simulink model "TesteMobotic_Initialization"  (R2024a)
settings: Solver=FixedStepDiscrete  StartTime=0.0  StopTime=inf  FixedStep=1e-3  RelTol=1e-3
model workspace (MAT data in the model file):
  RTK_health_condition = 30
  mdlWSDbList = ["tramontina_database_curtis.dbc" "tramontina_database_curtis_mesa.dbc" "tramontina_database_mobotic.dbc" "tramontina_database_nvidia.dbc" "tramontina_database_sick_modbus.dbc" "tramontina_database_xsens.dbc"]
undefined symbols (not defined in the file): Down, Pull
libraries: speedgoatlib_IO60X_IO69X x6, tramontina_database_curtislib x5, tramontina_database_curtis_mesalib x2, tramontina_database_moboticlib x2, speedgoatlib_IO691 x2, tramontina_database_nvidialib x1, canmsglib x1
settings Model: DataDictionary=configuration_dictionary.sldd  SimulationMode=external  ExtModeEnableFloating=off  Creator=matlab.cut  LastModifiedBy=matlab.cut
settings SolverCC: ConcurrentTasks=on  PositivePriorityOrder=on
settings OptimizationCC: BlockReduction=off  DefaultParameterBehavior=Inlined  OptimizeBlockIOStorage=off  EnhancedBackFolding=on  PassReuseOutputArgsThreshold=0  OptimizeBlockOrder=speed  DifferentSizesBufferReuse=on
settings DebuggingCC: UnderspecifiedInitializationDetection=Classic  MergeDetectMultiDrivingBlocksExec=none  TasksWithSamePriorityMsg=none  ParameterTunabilityLossMsg=error
settings HardwareCC: ProdBitPerLong=64  ProdLongLongMode=on  ProdHWDeviceType=Intel->x86-64 (Linux 64)
settings ModelReferenceCC: PropagateSignalLabelsOutOfModel=off
settings SFSimCC: MATLABDynamicMemAlloc=off
settings RTWCC: Description=Speedgoat Real-Time Target Machine  SystemTargetFile=speedgoat.tlc  TemplateMakefile=slrealtime_default_tmf  Toolchain=Simulink Real-Time Toolchain  BuildConfiguration=Faster Runs  CodeExecutionProfiling=on  TargetLang=C++  GPUComputeCapability=3.5
settings CodeAppCC: ForceParamTrailComments=on  MaxIdLength=127  OperatorAnnotations=on
settings SimulinkRealTimeTargetCC: InstructionSetFMA=off  LogToMDFFile=off

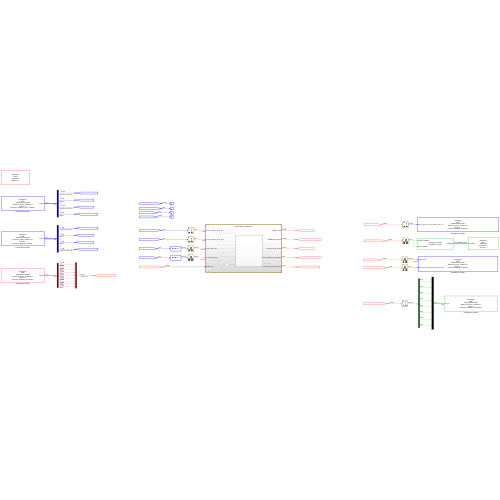
[thumbnail: Simulink's stored preview of the top-level diagram]
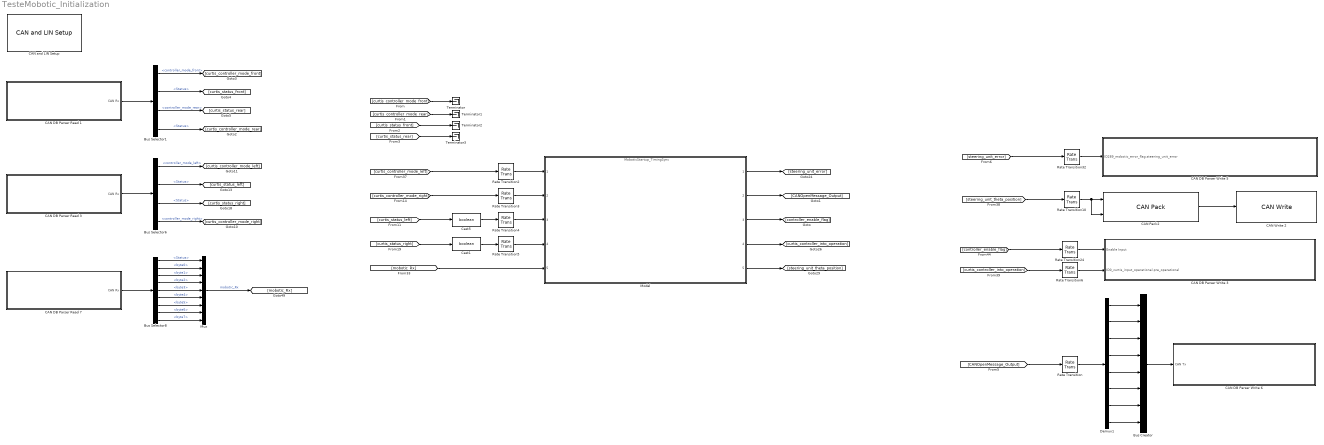
== system TesteMobotic_Initialization ==
  Bus Creator : BusCreator  Inputs=8
  Bus Selector1 : BusSelector  OutputSignals=ID1832_controller_status_RCUfront.controller_mode_front,ID1832_controller_status_RCUfront.MessageStatus.Status,ID1833_controller_status_RCUrear.controller_mode_rear,ID1833_controller_status_RCUrear.MessageStatus.Status
  Bus Selector6 : BusSelector  OutputSignals=ID1830_controller_status_left.controller_mode_left,ID1830_controller_status_left.MessageStatus.Status,ID1831_controller_status_right.MessageStatus.Status,ID1831_controller_status_right.controller_mode_right
  Bus Selector8 : BusSelector  OutputSignals=ID1459_feedback_word.MessageStatus.Status,ID1459_feedback_word.byte0,ID1459_feedback_word.byte1,ID1459_feedback_word.byte2,ID1459_feedback_word.byte3,ID1459_feedback_word.byte4,ID1459_feedback_word.byte5,ID1459_feedback_word.byte6,ID1459_feedback_word.byte7
  CAN DB Parser Read 1 : Subsystem
      settings: OpenFcn=sg_can.OpenFcnRead;
      mask Help: eval('sg.utils.help.show(''io_main/refentry_ref_can_ofa_parsing_read'');')
      mask Display: disp('Speedgoat\nIO691\nCAN DB Parser Read\nModule ID: IO691 - Module ID 1\nChannel:  1\ntramontina_database_curtis_mesa.dbc ');
  CAN DB Parser Read 3 : Subsystem
      settings: OpenFcn=sg_can.OpenFcnRead;
      mask Help: eval('sg.utils.help.show(''io_main/refentry_ref_can_ofa_parsing_read'');')
      mask Display: disp('Speedgoat\nIO691\nCAN DB Parser Read\nModule ID: IO691 - Module ID 1\nChannel:  1\ntramontina_database_curtis.dbc ');
  CAN DB Parser Read 7 : Subsystem
      settings: OpenFcn=sg_can.OpenFcnRead;
      mask Help: eval('sg.utils.help.show(''io_main/refentry_ref_can_ofa_parsing_read'');')
      mask Display: disp('Speedgoat\nIO691\nCAN DB Parser Read\nModule ID: IO691 - Module ID 1\nChannel:  1\ntramontina_database_mobotic.dbc ');
  CAN DB Parser Write 3 : Subsystem
      settings: OpenFcn=sg_can.OpenFcnWrite;
      mask Help: eval('sg.utils.help.show(''io_main/refentry_ref_can_ofa_parsing_write'');')
      mask Display: disp('Speedgoat\nIO691\nCAN DB Parser Write\nModule ID: IO691 - Module ID 1\nChannel:  1\ntramontina_database_curtis.dbc ');
  CAN DB Parser Write 5 : Subsystem
      settings: OpenFcn=sg_can.OpenFcnWrite;
      mask Help: eval('sg.utils.help.show(''io_main/refentry_ref_can_ofa_parsing_write'');')
      mask Display: disp('Speedgoat\nIO691\nCAN DB Parser Write\nModule ID: IO691 - Module ID 1\nChannel:  1\ntramontina_database_nvidia.dbc ');
  CAN DB Parser Write 6 : Subsystem
      settings: OpenFcn=sg_can.OpenFcnWrite;
      mask Help: eval('sg.utils.help.show(''io_main/refentry_ref_can_ofa_parsing_write'');')
      mask Display: disp('Speedgoat\nIO691\nCAN DB Parser Write\nModule ID: IO691 - Module ID 1\nChannel:  1\ntramontina_database_mobotic.dbc ');
  CAN Pack2 : canmsglib/CAN Pack  MsgList=(none)  MsgName=CAN Msg  MsgIDType=Standard (11-bit identifier)  MsgIdentifier=0x120  MsgLength=8  Remote=off  ApplyMinMax=off  BusOutput=on  SignalInfo={ 'position_feedback', '0', '32', 'LE', 'signed', 'Standard', '0', '1', '0', '-inf', 'inf'; 'pulse_feedback', '32', '32', 'LE', 'signed', 'Standard', '0', '1', '0', '-Inf', 'Inf' }
      settings: DataFormat=manually specified signals
  CAN Write 2 : speedgoatlib_IO691/CAN Write   moduleType=IO691  id=1  channel=1  canType=CAN (HS)  messageType=CAN (HS)  useBusIn=on  numOfMsg=1  enableInput=off  enableStatusPort=off  ts=10e-3  initValues=[691 1 0.01 0 1 1 0 1 0 1]
      settings: SourceProductName=IO691
  "CAN and LIN Setup " : speedgoatlib_IO691/CAN and LIN Setup   moduleInitValues="[691    1    1   -1   -1]"  id=1  moduleType=IO691  pciSlot=-1  canChn1=CAN (HS)  canChn2=Disabled  canChn3=Disabled  canChn4=Disabled  linChn1=Disabled  linChn2=Disabled  canInitStructArray=[]  canTermStructArray=[]  gpioChnx=Disabled  canChn1InitValues="[2   2   8   1  16   3  19   2   2   5   2   0]"  arbBdrChn1=500 kBaud  clockDividerChn1=Enable  arbManBdrChn1=[8,1,16,3]  fdBdrChn1=5.0 MBaud  fdManBdrChn1=[2,2,5,2]  termResistor1=off  canChn2InitValues="[1   0   2   8  31   8  19   2   2   5   2   0]"  arbBdrChn2=1.0 MBaud  clockDividerChn2=Enable  arbManBdrChn2=[2,8,31,8]  fdBdrChn2=5.0 MBaud  fdManBdrChn2=[2,2,5,2]  termResistor2=off  canChn3InitValues="[1   0   2   8  31   8  19   2   2   5   2   0]"  arbBdrChn3=1.0 MBaud  clockDividerChn3=Enable  arbManBdrChn3=[2,8,31,8]  fdBdrChn3=5.0 MBaud  fdManBdrChn3=[2,2,5,2]  termResistor3=off  canChn4InitValues="[1   0   2   8  31   8  19   2   2   5   2   0]"  arbBdrChn4=1.0 MBaud  clockDividerChn4=Enable  arbManBdrChn4=[2,8,31,8]  fdBdrChn4=5.0 MBaud  fdManBdrChn4=[2,2,5,2]  termResistor4=off  linChn1InitValues="[0  9600]"  linBtrChn1=9600  linChn2InitValues="[0  9600]"  linBtrChn2=9600  doInitTermStruct="[0  5  0  0  0]"  parDoChannels=[1 2]  parDoVoltage=5  parDoInitValues=0  parDoReset=1  parNumOfDoS=0  parDiChannels=[3 4]  parDiVoltage=5  parDiPull=Pull-Down
      settings: LibrarySourceBlock=speedgoatlib_IO602_IO691/CAN and LIN Setup
  Cast1 : DataTypeConversion  OutDataTypeStr=boolean  SaturateOnIntegerOverflow=off  RndMeth=Floor
  Cast5 : DataTypeConversion  OutDataTypeStr=boolean  SaturateOnIntegerOverflow=off  RndMeth=Floor
  Demux1 : Demux  Outputs=8
  Model : ModelReference  ModelNameDialog=MoboticStartup_TimingSync.slx  SimulationMode=Normal  ModelReferenceVersion=1.51
  Mux : Mux  Inputs=9
  Rate Transition{,2,6,10,24,32} (6 alike) : RateTransition
  Rate Transition3 : RateTransition  OutPortSampleTimeOpt=Inherit
  Rate Transition4 : RateTransition  OutPortSampleTimeOpt=Inherit
  Rate Transition5 : RateTransition  OutPortSampleTimeOpt=Inherit
  Terminator{,1..3} (4 alike) : Terminator
  wires:
  CAN Pack2/1 -> CAN Write 2/1
  Rate Transition6/1 -> CAN DB Parser Write 3/2(ID0_curtis_input_operational.pre_operational)
  [steering_unit_error] -> Rate Transition32/1
  Rate Transition10/1 -> CAN Pack2/2, CAN Pack2/1
  [curtis_controller_into_operation] -> Rate Transition6/1
  [steering_unit_theta_position] -> Rate Transition10/1
  [controller_enable_flag] -> Rate Transition24/1
  Rate Transition24/1 -> CAN DB Parser Write 3/1(Enable Input)
  Bus Selector6/2 -> [curtis_status_left]  "<Status>"
  Bus Selector8/7 -> Mux/7  "<byte5>"
  Bus Selector8/5 -> Mux/5  "<byte3>"
  Bus Selector8/1 -> Mux/1  "<Status>"
  Bus Selector8/2 -> Mux/2  "<byte0>"
  CAN DB Parser Read 3/1(CAN Rx) -> Bus Selector6/1
  CAN DB Parser Read 7/1(CAN Rx) -> Bus Selector8/1
  Bus Selector8/3 -> Mux/3  "<byte1>"
  Bus Selector8/6 -> Mux/6  "<byte4>"
  Mux/1 -> [mobotic_Rx]  "mobotic_Rx"
  Bus Selector8/8 -> Mux/8  "<byte6>"
  Bus Selector8/9 -> Mux/9  "<byte7>"
  Bus Selector6/4 -> [curtis_controller_mode_right]  "<controller_mode_right>"
  Bus Selector6/3 -> [curtis_status_right]  "<Status>"
  Bus Selector8/4 -> Mux/4  "<byte2>"
  Bus Selector6/1 -> [curtis_controller_mode_left]  "<controller_mode_left>"
  [curtis_controller_mode_left] -> Rate Transition2/1
  Cast5/1 -> Rate Transition4/1
  Cast1/1 -> Rate Transition5/1
  [curtis_controller_mode_right] -> Rate Transition3/1
  [curtis_status_left] -> Cast5/1
  [curtis_status_right] -> Cast1/1
  Rate Transition2/1 -> Model/1
  Rate Transition3/1 -> Model/2
  Rate Transition4/1 -> Model/3
  Rate Transition5/1 -> Model/4
  Rate Transition/1 -> Demux1/1
  Rate Transition32/1 -> CAN DB Parser Write 5/1(ID289_mobotic_error_flag.steering_unit_error)
  Model/2 -> [CANOpenMessage_Output]
  Model/1 -> [steering_unit_error]
  Model/5 -> [steering_unit_theta_position]
  Model/4 -> [curtis_controller_into_operation]
  Model/3 -> [controller_enable_flag]
  [CANOpenMessage_Output] -> Rate Transition/1
  Bus Selector1/1 -> [curtis_controller_mode_front]  "<controller_mode_front>"
  Bus Selector1/3 -> [curtis_status_rear]  "<controller_mode_rear>"
  Bus Selector1/4 -> [curtis_controller_mode_rear]  "<Status>"
  CAN DB Parser Read 1/1(CAN Rx) -> Bus Selector1/1
  Bus Selector1/2 -> [curtis_status_front]  "<Status>"
  [curtis_controller_mode_front] -> Terminator/1
  [curtis_status_front] -> Terminator2/1
  [curtis_controller_mode_rear] -> Terminator1/1
  [curtis_status_rear] -> Terminator3/1
  [mobotic_Rx] -> Model/5
  Demux1/1 -> Bus Creator/1
  Demux1/2 -> Bus Creator/2
  Demux1/3 -> Bus Creator/3
  Demux1/4 -> Bus Creator/4
  Demux1/5 -> Bus Creator/5
  Demux1/6 -> Bus Creator/6
  Demux1/7 -> Bus Creator/7
  Demux1/8 -> Bus Creator/8
  Bus Creator/1 -> CAN DB Parser Write 6/1(CAN Tx)

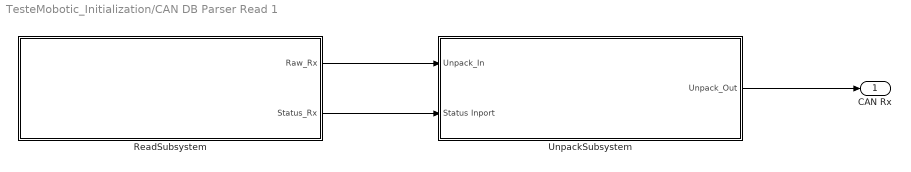
== system TesteMobotic_Initialization/CAN DB Parser Read 1 ==
  ReadSubsystem : Subsystem
  UnpackSubsystem : Subsystem
  CAN Rx : Outport
  wires:
  ReadSubsystem/1(Raw_Rx) -> UnpackSubsystem/1(Unpack_In)
  ReadSubsystem/2(Status_Rx) -> UnpackSubsystem/2(Status Inport)
  UnpackSubsystem/1(Unpack_Out) -> CAN Rx/1

== system TesteMobotic_Initialization/CAN DB Parser Read 3 ==
  ReadSubsystem : Subsystem
  UnpackSubsystem : Subsystem
  CAN Rx : Outport
  wires:
  ReadSubsystem/1(Raw_Rx) -> UnpackSubsystem/1(Unpack_In)
  ReadSubsystem/2(Status_Rx) -> UnpackSubsystem/2(Status Inport)
  UnpackSubsystem/1(Unpack_Out) -> CAN Rx/1

== system TesteMobotic_Initialization/CAN DB Parser Read 7 ==
  ReadSubsystem : Subsystem
  UnpackSubsystem : Subsystem
  CAN Rx : Outport
  wires:
  ReadSubsystem/1(Raw_Rx) -> UnpackSubsystem/1(Unpack_In)
  ReadSubsystem/2(Status_Rx) -> UnpackSubsystem/2(Status Inport)
  UnpackSubsystem/1(Unpack_Out) -> CAN Rx/1

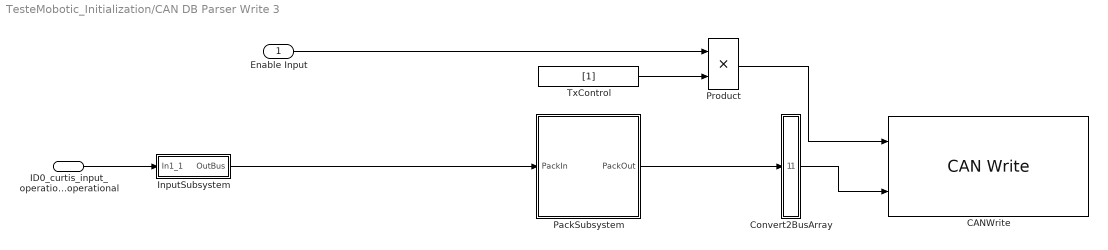
== system TesteMobotic_Initialization/CAN DB Parser Write 3 ==
  Enable Input : Inport  OutDataTypeStr=boolean
  ID0_curtis_input_operational.pre_operational : Inport  Port=2
  CANWrite : speedgoatlib_IO60X_IO69X/CAN/CAN Write   moduleType=IO691  id=1  channel=1  canType=CAN (HS)  messageType=CAN (HS)  useBusIn=on  numOfMsg=1  enableInput=on  enableStatusPort=off  ts=500e-3  initValues=[691 1 0.5 0 1 1 0 1 1 1]
  Convert2BusArray : Subsystem
  InputSubsystem : Subsystem
  PackSubsystem : Subsystem
  Product : Product  OutDataTypeStr=uint32
  TxControl : Constant  Value=[1]  OutDataTypeStr=uint32
  wires:
  PackSubsystem/1(PackOut) -> Convert2BusArray/1(InBus)
  Convert2BusArray/1(BusArrayOut) -> CANWrite/2
  Product/1 -> CANWrite/1
  TxControl/1 -> Product/2
  Enable Input/1 -> Product/1
  ID0_curtis_input_operational.pre_operational/1 -> InputSubsystem/1(In1_1)
  InputSubsystem/1(OutBus) -> PackSubsystem/1(PackIn)

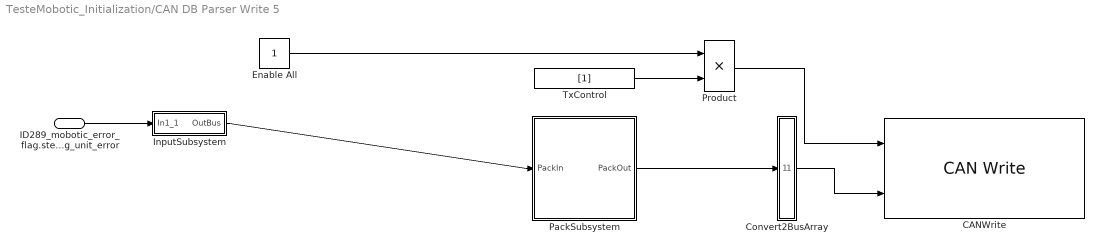
== system TesteMobotic_Initialization/CAN DB Parser Write 5 ==
  ID289_mobotic_error_flag.steering_unit_error : Inport
  CANWrite : speedgoatlib_IO60X_IO69X/CAN/CAN Write   moduleType=IO691  id=1  channel=1  canType=CAN (HS)  messageType=CAN (HS)  useBusIn=on  numOfMsg=1  enableInput=on  enableStatusPort=off  ts=500e-3  initValues=[691 1 0.5 0 1 1 0 1 1 1]
  Convert2BusArray : Subsystem
  Enable All : Constant  OutDataTypeStr=boolean
  InputSubsystem : Subsystem
  PackSubsystem : Subsystem
  Product : Product  OutDataTypeStr=uint32
  TxControl : Constant  Value=[1]  OutDataTypeStr=uint32
  wires:
  PackSubsystem/1(PackOut) -> Convert2BusArray/1(InBus)
  Convert2BusArray/1(BusArrayOut) -> CANWrite/2
  Product/1 -> CANWrite/1
  TxControl/1 -> Product/2
  Enable All/1 -> Product/1
  ID289_mobotic_error_flag.steering_unit_error/1 -> InputSubsystem/1(In1_1)
  InputSubsystem/1(OutBus) -> PackSubsystem/1(PackIn)

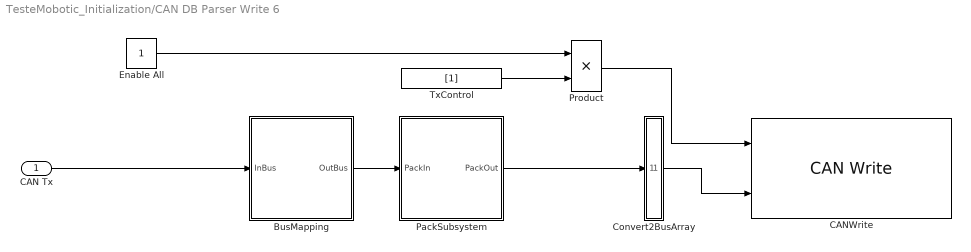
== system TesteMobotic_Initialization/CAN DB Parser Write 6 ==
  CAN Tx : Inport
  BusMapping : Subsystem
  CANWrite : speedgoatlib_IO60X_IO69X/CAN/CAN Write   moduleType=IO691  id=1  channel=1  canType=CAN (HS)  messageType=CAN (HS)  useBusIn=on  numOfMsg=1  enableInput=on  enableStatusPort=off  ts=10e-3  initValues=[691 1 0.01 0 1 1 0 1 1 1]
  Convert2BusArray : Subsystem
  Enable All : Constant  OutDataTypeStr=boolean
  PackSubsystem : Subsystem
  Product : Product  OutDataTypeStr=uint32
  TxControl : Constant  Value=[1]  OutDataTypeStr=uint32
  wires:
  PackSubsystem/1(PackOut) -> Convert2BusArray/1(InBus)
  Convert2BusArray/1(BusArrayOut) -> CANWrite/2
  Product/1 -> CANWrite/1
  TxControl/1 -> Product/2
  Enable All/1 -> Product/1
  CAN Tx/1 -> BusMapping/1(InBus)
  BusMapping/1(OutBus) -> PackSubsystem/1(PackIn)

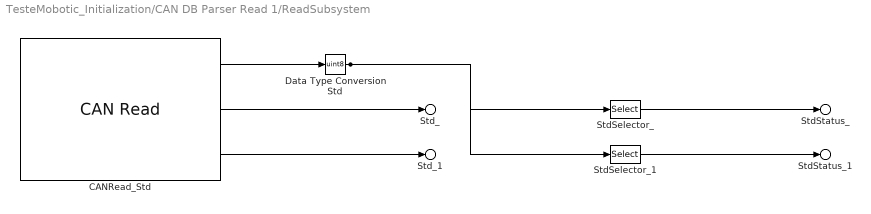
== system TesteMobotic_Initialization/CAN DB Parser Read 1/ReadSubsystem ==
  CANRead_Std : speedgoatlib_IO60X_IO69X/CAN/CAN Read   moduleType=IO691  id=1  channel=1  canType=CAN (HS)  messageType=CAN (HS)  useBusOut=on  HasMulRead=Specify by IDs  MsgIDlist="[1832  1833]"  isEFF=off  LabelInHex=off  enableInput=off  initValues=[691 1 0.05 0 1 1 0 1 2 0 2 1832 1833]  ts=50e-3
  Data Type ConversionStd : DataTypeConversion  OutDataTypeStr=uint8  SaturateOnIntegerOverflow=off  RndMeth=Floor
  StdSelector_ : Selector  IndexOptions=Index vector (dialog)  Indices=1  OutputSizes=1
  StdSelector_1 : Selector  IndexOptions=Index vector (dialog)  Indices=2  OutputSizes=1
  Std_ : Outport  PortName=Raw_Rx  Element=Std.ID1832
  Std_1 : Outport  PortName=Raw_Rx  Element=Std.ID1833
  StdStatus_ : Outport  Port=2  PortName=Status_Rx  Element=Std.ID1832
  StdStatus_1 : Outport  Port=2  PortName=Status_Rx  Element=Std.ID1833
  wires:
  CANRead_Std/1 -> Data Type ConversionStd/1
  CANRead_Std/2 -> Std_/1
  CANRead_Std/3 -> Std_1/1
  Data Type ConversionStd/1 -> StdSelector_/1, StdSelector_1/1
  StdSelector_/1 -> StdStatus_/1
  StdSelector_1/1 -> StdStatus_1/1

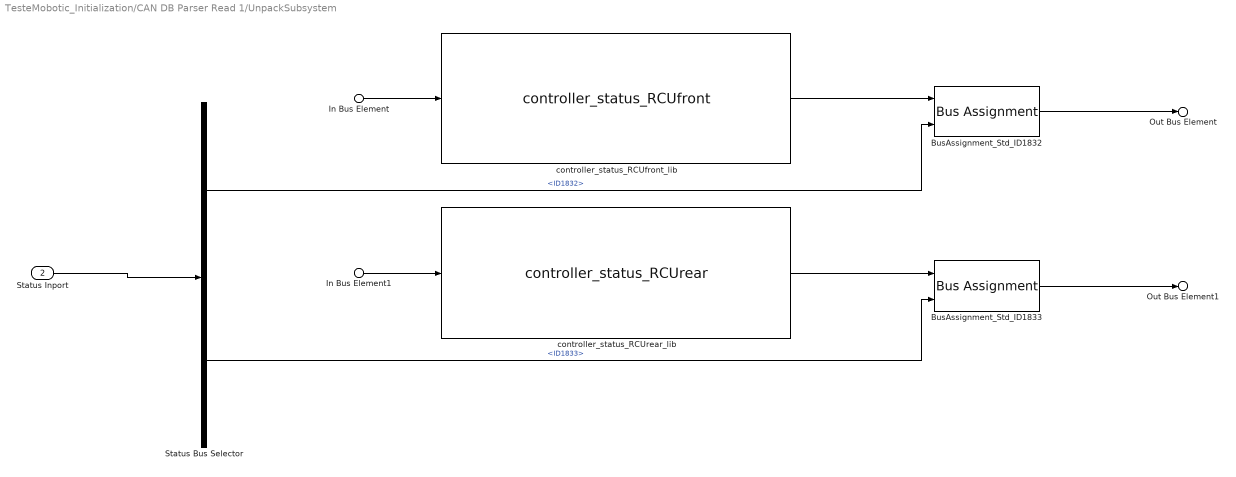
== system TesteMobotic_Initialization/CAN DB Parser Read 1/UnpackSubsystem ==
  In Bus Element : Inport  PortName=Unpack_In  Element=Std.ID1832
  In Bus Element1 : Inport  PortName=Unpack_In  Element=Std.ID1833
  Status Inport : Inport  Port=2
  BusAssignment_Std_ID1832 : BusAssignment  AssignedSignals=MessageStatus.Status
  BusAssignment_Std_ID1833 : BusAssignment  AssignedSignals=MessageStatus.Status
  Status Bus Selector : BusSelector  OutputSignals=Std.ID1832,Std.ID1833
  controller_status_RCUfront_lib : tramontina_database_curtis_mesalib/CAN unpack/controller_status_RCUfront  SystemSampleTime=-1  VariantActivationTime=update diagram  AllowFlexibleInterface=on  Latency=0  AutoFrameSizeCalculation=off
  controller_status_RCUrear_lib : tramontina_database_curtis_mesalib/CAN unpack/controller_status_RCUrear  SystemSampleTime=-1  VariantActivationTime=update diagram  AllowFlexibleInterface=on  Latency=0  AutoFrameSizeCalculation=off
  Out Bus Element : Outport  PortName=Unpack_Out  Element=ID1832_controller_status_RCUfront
  Out Bus Element1 : Outport  PortName=Unpack_Out  Element=ID1833_controller_status_RCUrear
  wires:
  In Bus Element/1 -> controller_status_RCUfront_lib/1
  controller_status_RCUfront_lib/1 -> BusAssignment_Std_ID1832/1
  BusAssignment_Std_ID1832/1 -> Out Bus Element/1
  In Bus Element1/1 -> controller_status_RCUrear_lib/1
  controller_status_RCUrear_lib/1 -> BusAssignment_Std_ID1833/1
  BusAssignment_Std_ID1833/1 -> Out Bus Element1/1
  Status Inport/1 -> Status Bus Selector/1
  Status Bus Selector/1 -> BusAssignment_Std_ID1832/2  "<ID1832>"
  Status Bus Selector/2 -> BusAssignment_Std_ID1833/2  "<ID1833>"

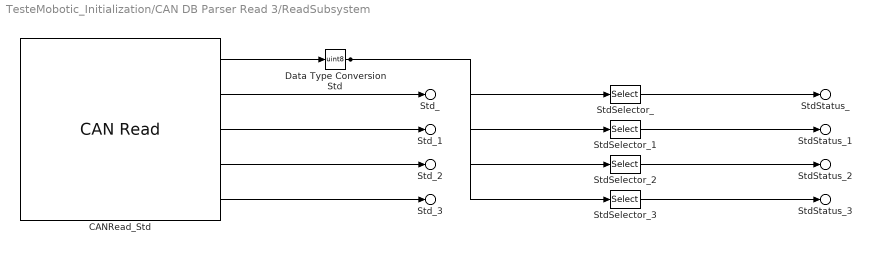
== system TesteMobotic_Initialization/CAN DB Parser Read 3/ReadSubsystem ==
  CANRead_Std : speedgoatlib_IO60X_IO69X/CAN/CAN Read   moduleType=IO691  id=1  channel=1  canType=CAN (HS)  messageType=CAN (HS)  useBusOut=on  HasMulRead=Specify by IDs  MsgIDlist="[422   423  1830  1831]"  isEFF=off  LabelInHex=off  enableInput=off  initValues=[691 1 0.05 0 1 1 0 1 2 0 4 422 423 1830 1831]  ts=50e-3
  Data Type ConversionStd : DataTypeConversion  OutDataTypeStr=uint8  SaturateOnIntegerOverflow=off  RndMeth=Floor
  StdSelector_ : Selector  IndexOptions=Index vector (dialog)  Indices=1  OutputSizes=1
  StdSelector_1 : Selector  IndexOptions=Index vector (dialog)  Indices=2  OutputSizes=1
  StdSelector_2 : Selector  IndexOptions=Index vector (dialog)  Indices=3  OutputSizes=1
  StdSelector_3 : Selector  IndexOptions=Index vector (dialog)  Indices=4  OutputSizes=1
  Std_ : Outport  PortName=Raw_Rx  Element=Std.ID422
  Std_1 : Outport  PortName=Raw_Rx  Element=Std.ID423
  Std_2 : Outport  PortName=Raw_Rx  Element=Std.ID1830
  Std_3 : Outport  PortName=Raw_Rx  Element=Std.ID1831
  StdStatus_ : Outport  Port=2  PortName=Status_Rx  Element=Std.ID422
  StdStatus_1 : Outport  Port=2  PortName=Status_Rx  Element=Std.ID423
  StdStatus_2 : Outport  Port=2  PortName=Status_Rx  Element=Std.ID1830
  StdStatus_3 : Outport  Port=2  PortName=Status_Rx  Element=Std.ID1831
  wires:
  CANRead_Std/1 -> Data Type ConversionStd/1
  CANRead_Std/2 -> Std_/1
  CANRead_Std/3 -> Std_1/1
  CANRead_Std/4 -> Std_2/1
  CANRead_Std/5 -> Std_3/1
  Data Type ConversionStd/1 -> StdSelector_/1, StdSelector_1/1, StdSelector_2/1, StdSelector_3/1
  StdSelector_/1 -> StdStatus_/1
  StdSelector_1/1 -> StdStatus_1/1
  StdSelector_2/1 -> StdStatus_2/1
  StdSelector_3/1 -> StdStatus_3/1

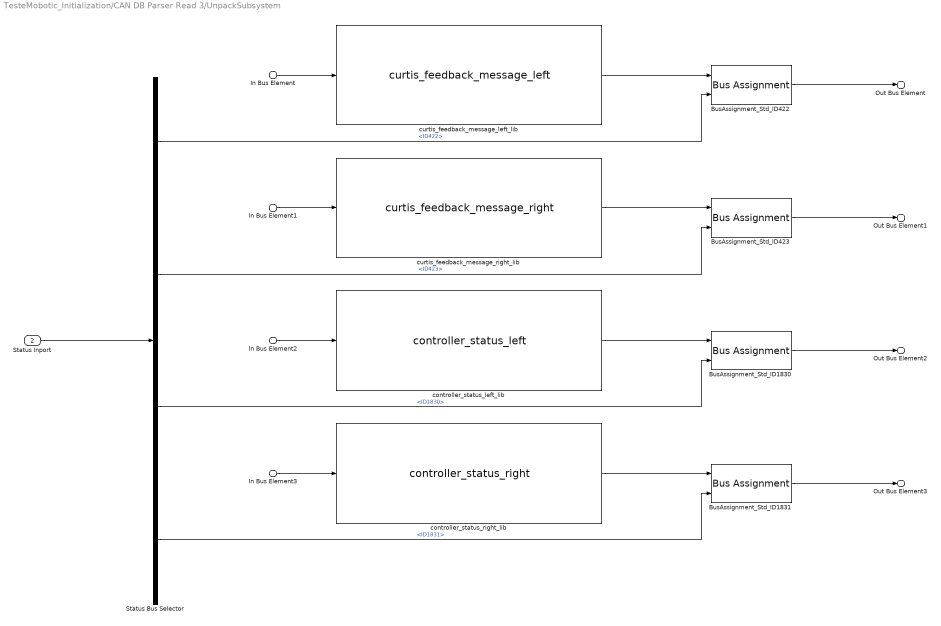
== system TesteMobotic_Initialization/CAN DB Parser Read 3/UnpackSubsystem ==
  In Bus Element : Inport  PortName=Unpack_In  Element=Std.ID422
  In Bus Element1 : Inport  PortName=Unpack_In  Element=Std.ID423
  In Bus Element2 : Inport  PortName=Unpack_In  Element=Std.ID1830
  In Bus Element3 : Inport  PortName=Unpack_In  Element=Std.ID1831
  Status Inport : Inport  Port=2
  BusAssignment_Std_ID{422..423,1830..1831} (4 alike) : BusAssignment  AssignedSignals=MessageStatus.Status
  Status Bus Selector : BusSelector  OutputSignals=Std.ID422,Std.ID423,Std.ID1830,Std.ID1831
  controller_status_left_lib : tramontina_database_curtislib/CAN unpack/controller_status_left  SystemSampleTime=-1  VariantActivationTime=update diagram  AllowFlexibleInterface=on  Latency=0  AutoFrameSizeCalculation=off
  controller_status_right_lib : tramontina_database_curtislib/CAN unpack/controller_status_right  SystemSampleTime=-1  VariantActivationTime=update diagram  AllowFlexibleInterface=on  Latency=0  AutoFrameSizeCalculation=off
  curtis_feedback_message_left_lib : tramontina_database_curtislib/CAN unpack/curtis_feedback_message_left  SystemSampleTime=-1  VariantActivationTime=update diagram  AllowFlexibleInterface=on  Latency=0  AutoFrameSizeCalculation=off
  curtis_feedback_message_right_lib : tramontina_database_curtislib/CAN unpack/curtis_feedback_message_right  SystemSampleTime=-1  VariantActivationTime=update diagram  AllowFlexibleInterface=on  Latency=0  AutoFrameSizeCalculation=off
  Out Bus Element : Outport  PortName=Unpack_Out  Element=ID422_curtis_feedback_message_left
  Out Bus Element1 : Outport  PortName=Unpack_Out  Element=ID423_curtis_feedback_message_right
  Out Bus Element2 : Outport  PortName=Unpack_Out  Element=ID1830_controller_status_left
  Out Bus Element3 : Outport  PortName=Unpack_Out  Element=ID1831_controller_status_right
  wires:
  In Bus Element/1 -> curtis_feedback_message_left_lib/1
  curtis_feedback_message_left_lib/1 -> BusAssignment_Std_ID422/1
  BusAssignment_Std_ID422/1 -> Out Bus Element/1
  In Bus Element1/1 -> curtis_feedback_message_right_lib/1
  curtis_feedback_message_right_lib/1 -> BusAssignment_Std_ID423/1
  BusAssignment_Std_ID423/1 -> Out Bus Element1/1
  In Bus Element2/1 -> controller_status_left_lib/1
  controller_status_left_lib/1 -> BusAssignment_Std_ID1830/1
  BusAssignment_Std_ID1830/1 -> Out Bus Element2/1
  In Bus Element3/1 -> controller_status_right_lib/1
  controller_status_right_lib/1 -> BusAssignment_Std_ID1831/1
  BusAssignment_Std_ID1831/1 -> Out Bus Element3/1
  Status Inport/1 -> Status Bus Selector/1
  Status Bus Selector/1 -> BusAssignment_Std_ID422/2  "<ID422>"
  Status Bus Selector/2 -> BusAssignment_Std_ID423/2  "<ID423>"
  Status Bus Selector/3 -> BusAssignment_Std_ID1830/2  "<ID1830>"
  Status Bus Selector/4 -> BusAssignment_Std_ID1831/2  "<ID1831>"

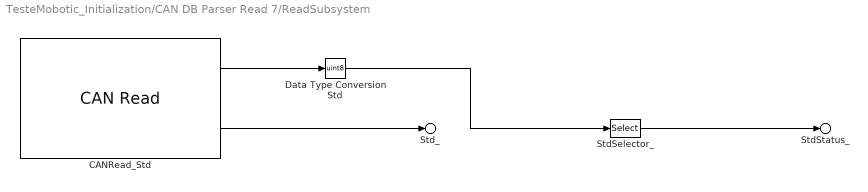
== system TesteMobotic_Initialization/CAN DB Parser Read 7/ReadSubsystem ==
  CANRead_Std : speedgoatlib_IO60X_IO69X/CAN/CAN Read   moduleType=IO691  id=1  channel=1  canType=CAN (HS)  messageType=CAN (HS)  useBusOut=on  HasMulRead=Specify by IDs  MsgIDlist=[1459]  isEFF=off  LabelInHex=off  enableInput=off  initValues=[691 1 0.001 0 1 1 0 1 2 0 1 1459]  ts=1e-3
  Data Type ConversionStd : DataTypeConversion  OutDataTypeStr=uint8  SaturateOnIntegerOverflow=off  RndMeth=Floor
  StdSelector_ : Selector  IndexOptions=Index vector (dialog)  Indices=1  OutputSizes=1
  Std_ : Outport  PortName=Raw_Rx  Element=Std.ID1459
  StdStatus_ : Outport  Port=2  PortName=Status_Rx  Element=Std.ID1459
  wires:
  CANRead_Std/1 -> Data Type ConversionStd/1
  CANRead_Std/2 -> Std_/1
  Data Type ConversionStd/1 -> StdSelector_/1
  StdSelector_/1 -> StdStatus_/1

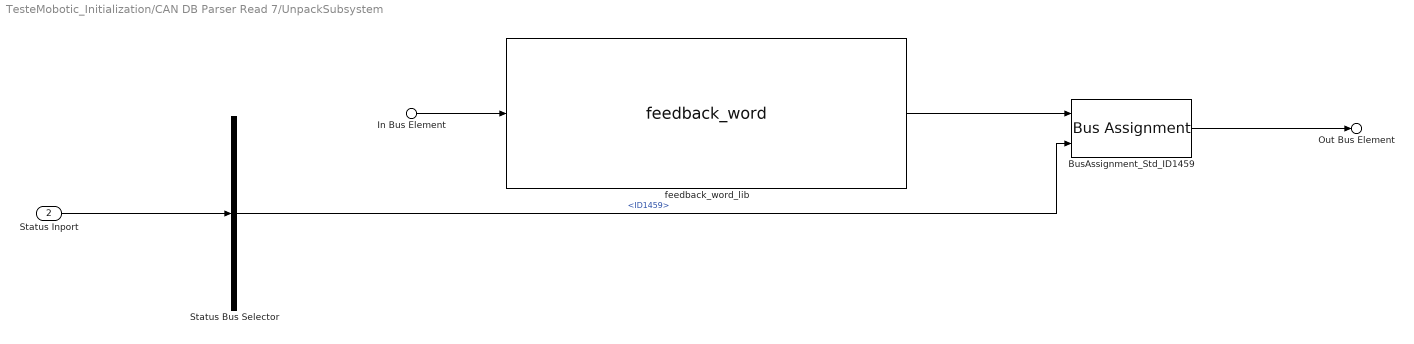
== system TesteMobotic_Initialization/CAN DB Parser Read 7/UnpackSubsystem ==
  In Bus Element : Inport  PortName=Unpack_In  Element=Std.ID1459
  Status Inport : Inport  Port=2
  BusAssignment_Std_ID1459 : BusAssignment  AssignedSignals=MessageStatus.Status
  Status Bus Selector : BusSelector  OutputSignals=Std.ID1459
  feedback_word_lib : tramontina_database_moboticlib/CAN unpack/feedback_word  SystemSampleTime=-1  VariantActivationTime=update diagram  AllowFlexibleInterface=on  Latency=0  AutoFrameSizeCalculation=off
  Out Bus Element : Outport  PortName=Unpack_Out  Element=ID1459_feedback_word
  wires:
  In Bus Element/1 -> feedback_word_lib/1
  feedback_word_lib/1 -> BusAssignment_Std_ID1459/1
  BusAssignment_Std_ID1459/1 -> Out Bus Element/1
  Status Inport/1 -> Status Bus Selector/1
  Status Bus Selector/1 -> BusAssignment_Std_ID1459/2  "<ID1459>"

== system TesteMobotic_Initialization/CAN DB Parser Write 3/Convert2BusArray ==
  In1 : Inport  PortName=InBus  Element=ID0_curtis_input_operational
  BusArray : Concatenate  NumInputs=1
  BusArrayOut : Outport
  wires:
  In1/1 -> BusArray/1
  BusArray/1 -> BusArrayOut/1

== system TesteMobotic_Initialization/CAN DB Parser Write 3/InputSubsystem ==
  In1_1 : Inport
  ID0_curtis_input_operational.pre_operational : Outport  PortName=OutBus  Element=ID0_curtis_input_operational.pre_operational
  wires:
  In1_1/1 -> ID0_curtis_input_operational.pre_operational/1

== system TesteMobotic_Initialization/CAN DB Parser Write 3/PackSubsystem ==
  In Bus Element : Inport  PortName=PackIn  Element=ID0_curtis_input_operational
  curtis_input_operational_lib : tramontina_database_curtislib/CAN pack/curtis_input_operational  SystemSampleTime=-1  VariantActivationTime=update diagram  AllowFlexibleInterface=on  Latency=0  AutoFrameSizeCalculation=off
  In Bus Element1 : Outport  PortName=PackOut  Element=ID0_curtis_input_operational
  wires:
  In Bus Element/1 -> curtis_input_operational_lib/1
  curtis_input_operational_lib/1 -> In Bus Element1/1

== system TesteMobotic_Initialization/CAN DB Parser Write 5/Convert2BusArray ==
  In1 : Inport  PortName=InBus  Element=ID289_mobotic_error_flag
  BusArray : Concatenate  NumInputs=1
  BusArrayOut : Outport
  wires:
  In1/1 -> BusArray/1
  BusArray/1 -> BusArrayOut/1

== system TesteMobotic_Initialization/CAN DB Parser Write 5/InputSubsystem ==
  In1_1 : Inport
  ID289_mobotic_error_flag.steering_unit_error : Outport  PortName=OutBus  Element=ID289_mobotic_error_flag.steering_unit_error
  wires:
  In1_1/1 -> ID289_mobotic_error_flag.steering_unit_error/1

== system TesteMobotic_Initialization/CAN DB Parser Write 5/PackSubsystem ==
  In Bus Element : Inport  PortName=PackIn  Element=ID289_mobotic_error_flag
  mobotic_error_flag_lib : tramontina_database_nvidialib/CAN pack/mobotic_error_flag  SystemSampleTime=-1  VariantActivationTime=update diagram  AllowFlexibleInterface=on  Latency=0  AutoFrameSizeCalculation=off
  In Bus Element1 : Outport  PortName=PackOut  Element=ID289_mobotic_error_flag
  wires:
  In Bus Element/1 -> mobotic_error_flag_lib/1
  mobotic_error_flag_lib/1 -> In Bus Element1/1

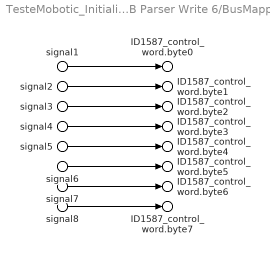
== system TesteMobotic_Initialization/CAN DB Parser Write 6/BusMapping ==
  signal1 : Inport  PortName=InBus  Element=signal1
  signal2 : Inport  PortName=InBus  Element=signal2
  signal3 : Inport  PortName=InBus  Element=signal3
  signal4 : Inport  PortName=InBus  Element=signal4
  signal5 : Inport  PortName=InBus  Element=signal5
  signal6 : Inport  PortName=InBus  Element=signal6
  signal7 : Inport  PortName=InBus  Element=signal7
  signal8 : Inport  PortName=InBus  Element=signal8
  ID1587_control_word.byte0 : Outport  PortName=OutBus  Element=ID1587_control_word.byte0
  ID1587_control_word.byte1 : Outport  PortName=OutBus  Element=ID1587_control_word.byte1
  ID1587_control_word.byte2 : Outport  PortName=OutBus  Element=ID1587_control_word.byte2
  ID1587_control_word.byte3 : Outport  PortName=OutBus  Element=ID1587_control_word.byte3
  ID1587_control_word.byte4 : Outport  PortName=OutBus  Element=ID1587_control_word.byte4
  ID1587_control_word.byte5 : Outport  PortName=OutBus  Element=ID1587_control_word.byte5
  ID1587_control_word.byte6 : Outport  PortName=OutBus  Element=ID1587_control_word.byte6
  ID1587_control_word.byte7 : Outport  PortName=OutBus  Element=ID1587_control_word.byte7
  wires:
  signal1/1 -> ID1587_control_word.byte0/1
  signal2/1 -> ID1587_control_word.byte1/1
  signal3/1 -> ID1587_control_word.byte2/1
  signal4/1 -> ID1587_control_word.byte3/1
  signal5/1 -> ID1587_control_word.byte4/1
  signal6/1 -> ID1587_control_word.byte5/1
  signal7/1 -> ID1587_control_word.byte6/1
  signal8/1 -> ID1587_control_word.byte7/1

== system TesteMobotic_Initialization/CAN DB Parser Write 6/Convert2BusArray ==
  In1 : Inport  PortName=InBus  Element=ID1587_control_word
  BusArray : Concatenate  NumInputs=1
  BusArrayOut : Outport
  wires:
  In1/1 -> BusArray/1
  BusArray/1 -> BusArrayOut/1

== system TesteMobotic_Initialization/CAN DB Parser Write 6/PackSubsystem ==
  In Bus Element : Inport  PortName=PackIn  Element=ID1587_control_word
  control_word_lib : tramontina_database_moboticlib/CAN pack/control_word  SystemSampleTime=-1  VariantActivationTime=update diagram  AllowFlexibleInterface=on  Latency=0  AutoFrameSizeCalculation=off
  In Bus Element1 : Outport  PortName=PackOut  Element=ID1587_control_word
  wires:
  In Bus Element/1 -> control_word_lib/1
  control_word_lib/1 -> In Bus Element1/1
